simulink model "Test_Configuration"  (R2016b)
settings: Solver=FixedStepDiscrete  StartTime=0.0  StopTime=inf  FixedStep=TestCfg.tiSimnTiStep_C.Value  RelTol=1e-3  EnableMultiTasking=on
InitFcn:
  | % Call parameters initialization function
  | % run optiTruck_init_sim.m;
StopFcn:
  | %optiTruck_post_sim;
  | %optiTruck_plot_sim;
settings Model: Creator=engin  LastModifiedBy=bunver
settings DataIOCC: SaveFormat=StructureWithTime  SaveOutput=off  DSMLogging=off  VisualizeSimOutput=off  SaveTime=off  SignalLoggingName=Results
settings OptimizationCC: BlockReduction=off  ConditionallyExecuteInputs=off  LifeSpan=inf
settings DebuggingCC: AllowSymbolicDim=off  SFUnexpectedBacktrackingDiag=warning  SFNoUnconditionalDefaultTransitionDiag=warning  SFExecutionAtInitializationDiag=none
settings ModelReferenceCC: ModelReferenceNumInstancesAllowed=Single  PropagateSignalLabelsOutOfModel=off
settings GRTTargetCC: TargetLangStandard=C89/C90 (ANSI)
settings ConfigComp: CovMetricSettings=dw  CovHtmlReporting=on  CovSaveCumulativeToWorkspaceVar=on  CovSaveSingleToWorkspaceVar=on  CovExternalEMLEnable=off

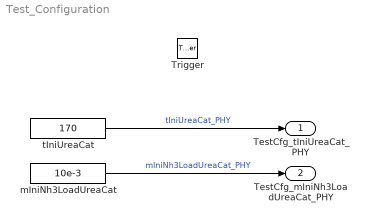
== system Test_Configuration ==
  Trigger : TriggerPort  TriggerType=function-call  VariantControl=Variant  PortDimensions=1
  mIniNh3LoadUreaCat : Constant  Value=10e-3  SampleTime=-1
  tIniUreaCat : Constant  Value=170  SampleTime=-1
  TestCfg_tIniUreaCat_PHY : Outport
  TestCfg_mIniNh3LoadUreaCat_PHY : Outport  Port=2
  wires:
  tIniUreaCat/1 -> TestCfg_tIniUreaCat_PHY/1  "tIniUreaCat_PHY"
  mIniNh3LoadUreaCat/1 -> TestCfg_mIniNh3LoadUreaCat_PHY/1  "mIniNh3LoadUreaCat_PHY"
